simulink model "Simulation"  (R2025b)
settings: Solver=ode4  StartTime=0.0  StopTime=Tfin  FixedStep=Ts  RelTol=1e-3
undefined symbols (not defined in the file): period, radius, ReferenceTypeNumber, speed, Ts
settings Model: SimulationMode=accelerator  SILPILSystemUnderTest=refmodels  CodeVerificationMode=processor-in-the-loop (pil)  Creator=baldo  LastModifiedBy=robyd
settings OptimizationCC: DefaultParameterBehavior=Inlined  EnhancedBackFolding=on  PassReuseOutputArgsThreshold=0.0  OptimizeBlockOrder=speed  DifferentSizesBufferReuse=on  OptimizationCustomize=off
settings DebuggingCC: ParameterTunabilityLossMsg=error  UnconnectedInputMsg=warning  UnconnectedOutputMsg=warning  UnconnectedLineMsg=warning
settings ModelReferenceCC: EnableRefExpFcnMdlSchedulingChecks=on  PropagateVarSize=During execution
settings SFSimCC: MATLABDynamicMemAlloc=off
settings RTWCC: GPUComputeCapability=3.5  DLArmComputeVersion=19.05
settings CodeAppCC: ForceParamTrailComments=on  OperatorAnnotations=on

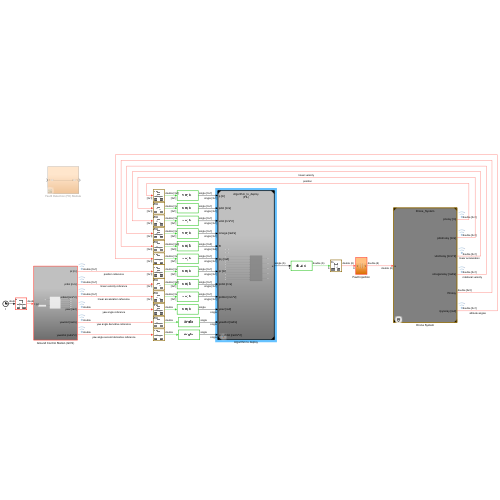
[thumbnail: Simulink's stored preview of the top-level diagram]
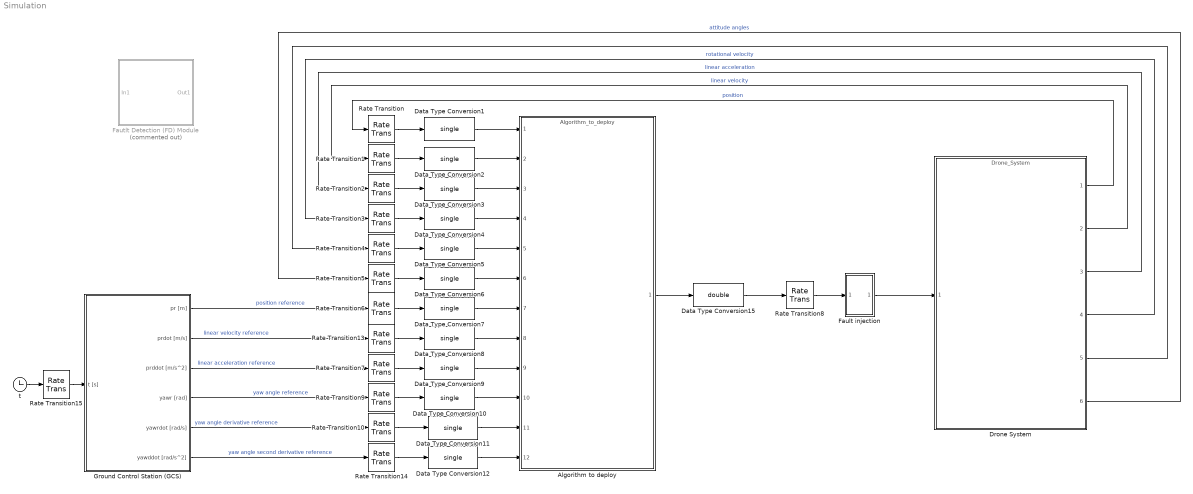
== system Simulation ==
  Algorithm to deploy : ModelReference  ModelNameDialog=Algorithm_to_deploy  SimulationMode=Processor-in-the-loop (PIL)  ModelReferenceVersion=9.14
  Data Type Conversion{1..12} (12 alike) : DataTypeConversion  OutDataTypeStr=single  SaturateOnIntegerOverflow=off  RndMeth=Floor
  Data Type Conversion15 : DataTypeConversion  OutDataTypeStr=double  SaturateOnIntegerOverflow=off  RndMeth=Floor
  Drone System : ModelReference  ModelNameDialog=Drone_System  ModelReferenceVersion=9.10  CopyOfModelProtected=on
  Fault injection : Subsystem
  Fautlt Detection (FD) Module : Subsystem  Commented=on
  Ground Control Station (GCS) : Subsystem
  Rate Transition{,1..7,9..10,13..14} (12 alike) : RateTransition  OutPortSampleTime=Ts_hw
  Rate Transition15 : RateTransition  OutPortSampleTime=Ts
  Rate Transition8 : RateTransition  OutPortSampleTime=Ts
  t : Clock
  wires:
  Algorithm to deploy/1 -> Data Type Conversion15/1
  Rate Transition/1 -> Data Type Conversion1/1
  Rate Transition1/1 -> Data Type Conversion2/1
  Rate Transition2/1 -> Data Type Conversion3/1
  Rate Transition3/1 -> Data Type Conversion4/1
  Rate Transition4/1 -> Data Type Conversion5/1
  Rate Transition5/1 -> Data Type Conversion6/1
  Rate Transition6/1 -> Data Type Conversion7/1
  Rate Transition13/1 -> Data Type Conversion8/1
  Rate Transition7/1 -> Data Type Conversion9/1
  Rate Transition9/1 -> Data Type Conversion10/1
  Rate Transition10/1 -> Data Type Conversion11/1
  Rate Transition14/1 -> Data Type Conversion12/1
  t/1 -> Rate Transition15/1
  Ground Control Station (GCS)/1(pr [m]) -> Rate Transition6/1  "position reference"
  Ground Control Station (GCS)/2(prdot [m/s]) -> Rate Transition13/1  "linear velocity reference"
  Ground Control Station (GCS)/3(prddot [m/s^2]) -> Rate Transition7/1  "linear acceleration reference"
  Ground Control Station (GCS)/4(yawr [rad]) -> Rate Transition9/1  "yaw angle reference"
  Ground Control Station (GCS)/5(yawrdot [rad/s]) -> Rate Transition10/1  "yaw angle derivative reference"
  Ground Control Station (GCS)/6(yawddot [rad/s^2]) -> Rate Transition14/1  "yaw angle second derivative reference"
  Data Type Conversion1/1 -> Algorithm to deploy/1
  Data Type Conversion2/1 -> Algorithm to deploy/2
  Data Type Conversion3/1 -> Algorithm to deploy/3
  Data Type Conversion4/1 -> Algorithm to deploy/4
  Data Type Conversion5/1 -> Algorithm to deploy/5
  Data Type Conversion6/1 -> Algorithm to deploy/6
  Data Type Conversion7/1 -> Algorithm to deploy/7
  Data Type Conversion8/1 -> Algorithm to deploy/8
  Data Type Conversion9/1 -> Algorithm to deploy/9
  Data Type Conversion10/1 -> Algorithm to deploy/10
  Data Type Conversion11/1 -> Algorithm to deploy/11
  Data Type Conversion12/1 -> Algorithm to deploy/12
  Data Type Conversion15/1 -> Rate Transition8/1
  Rate Transition15/1 -> Ground Control Station (GCS)/1(t [s])
  Drone System/1 -> Rate Transition/1  "position"
  Drone System/2 -> Rate Transition1/1  "linear velocity"
  Drone System/3 -> Rate Transition2/1  "linear acceleration"
  Drone System/4 -> Rate Transition3/1  "rotational velocity"
  Drone System/5 -> Rate Transition4/1
  Drone System/6 -> Rate Transition5/1  "attitude angles"
  Rate Transition8/1 -> Fault injection/1(In1)
  Fault injection/1(Out1) -> Drone System/1

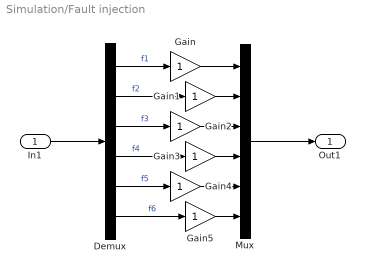
== system Simulation/Fault injection ==
  In1 : Inport
  Demux : Demux  Outputs=6
  Gain{,1..5} (6 alike) : Gain
  Mux : Mux  Inputs=6
  Out1 : Outport
  wires:
  Demux/2 -> Gain1/1  "f2"
  Demux/1 -> Gain/1  "f1"
  Demux/5 -> Gain4/1  "f5"
  Demux/3 -> Gain2/1  "f3"
  Gain5/1 -> Mux/6
  Gain2/1 -> Mux/3
  In1/1 -> Demux/1
  Mux/1 -> Out1/1
  Gain/1 -> Mux/1
  Demux/4 -> Gain3/1  "f4"
  Gain1/1 -> Mux/2
  Demux/6 -> Gain5/1  "f6"
  Gain4/1 -> Mux/5
  Gain3/1 -> Mux/4

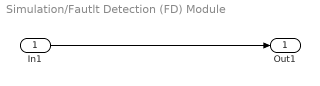
== system Simulation/Fautlt Detection (FD) Module ==
  In1 : Inport
  Out1 : Outport
  wires:
  In1/1 -> Out1/1

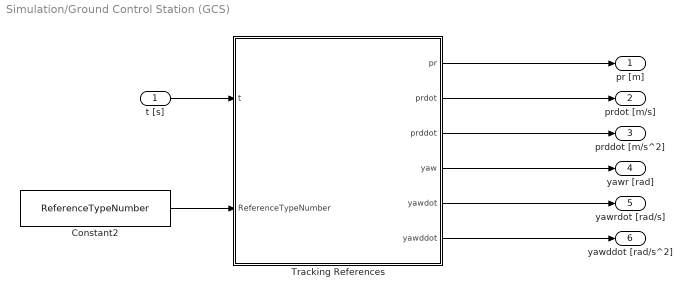
== system Simulation/Ground Control Station (GCS) ==
  t [s] : Inport
  Constant2 : Constant  Value=ReferenceTypeNumber  SampleTime=Ts
  Tracking References : MATLAB Function  TreatAsAtomicUnit=on
  pr [m] : Outport
  prdot [m/s] : Outport  Port=2
  prddot [m/s^2] : Outport  Port=3
  yawr [rad] : Outport  Port=4
  yawrdot [rad/s] : Outport  Port=5
  yawddot [rad/s^2] : Outport  Port=6
  wires:
  Tracking References/5(yawdot) -> yawrdot [rad/s]/1
  Tracking References/6(yawddot) -> yawddot [rad/s^2]/1
  Tracking References/3(prddot) -> prddot [m/s^2]/1
  Tracking References/2(prdot) -> prdot [m/s]/1
  Tracking References/4(yaw) -> yawr [rad]/1
  Tracking References/1(pr) -> pr [m]/1
  t [s]/1 -> Tracking References/1(t)
  Constant2/1 -> Tracking References/2(ReferenceTypeNumber)

== matlab function Simulation/Ground Control Station (GCS)/Tracking References ==
  data: t input; pr output; prdot output; prddot output; yaw output; speed parameter; period parameter; radius parameter; ReferenceTypeNumber input; yawdot output; yawddot output
function [pr,prdot,prddot,yaw,yawdot,yawddot] = RefGen(t, speed, period, radius, ReferenceTypeNumber)

% Extended references with derivatives
% prExtended = [pr prdot prddot] in R^{3x3}
% yawExtended = [yaw yawdot yawddot] in R^{1x3}

r = radius;
T = period;
v = speed;

if ReferenceTypeNumber == 0  % Origin

    prExtended = [NullWaveExtended(t); NullWaveExtended(t); NullWaveExtended(t)];
    yawExtended = NullWaveExtended(t);

elseif ReferenceTypeNumber == 1  % Constant speed in direction of xE

    prExtended = [speed*rampExtended(t); NullWaveExtended(t); NullWaveExtended(t)];
    yawExtended = NullWaveExtended(t);

elseif ReferenceTypeNumber == 2  % Constant speed in direction of yE

    prExtended = [NullWaveExtended(t); speed*rampExtended(t); NullWaveExtended(t)];
    yawExtended = NullWaveExtended(t);

elseif ReferenceTypeNumber == 3  % Constant speed in direction of -zE

    prExtended = [NullWaveExtended(t); NullWaveExtended(t); -speed*rampExtended(t)];
    yawExtended = NullWaveExtended(t);

elseif ReferenceTypeNumber == 4  % Ascending spiral
    
    pulsation = 2*pi/period;
    prExtended = [radius*CosineWaveExtended(t,pulsation)-radius*[1 0 0]; radius*SineWaveExtended(t,pulsation); -speed*rampExtended(t)];
    yawExtended = zeros(1,3);

    % omegayaw = 2*pi/5;
    % yawExtended = SineWaveExtended(t,omegayaw);

elseif ReferenceTypeNumber == 5  % Ascending 8-shape

    pulsation = 2*pi/period;
    prExtended = [radius*CosineWaveExtended(t,pulsation)-radius*[1 0 0]; 0.5*radius*SineWaveExtended(t,2*pulsation); -speed*rampExtended(t)];
    yawExtended = zeros(1,3);

elseif ReferenceTypeNumber == 6  % Square around e3

    prExtended = zeros(3,3);
    yawExtended = zeros(1,3);
    
    % L = 2*r;
    % t2 = mod(t,T);
    % pr = (4*L/T)*[ramp(t2)-ramp(t2-T/4)-ramp(t2-T/2)+ramp(t2-3*T/4); ramp(t2-T/4)-ramp(t2-T/2)-ramp(t2-3*T/4)+ramp(t2-T); -v*t];
    % psir = 0;
elseif ReferenceTypeNumber == 7

    prExtended = [SawtoothWaveExtended(t,20); NullWaveExtended(t); NullWaveExtended(t)];
    yawExtended = zeros(1,3);

elseif ReferenceTypeNumber == 8
    
    prExtended = [NullWaveExtended(t); NullWaveExtended(t); -SawtoothWave(t,20) 0 0];
    yawExtended = zeros(1,3);

elseif ReferenceTypeNumber == 9  % Descending spiral
    
    pulsation = 2*pi/period;
    prExtended = [radius*CosineWaveExtended(t,pulsation)-radius*[1 0 0]; 0.5*radius*SineWaveExtended(t,2*pulsation); (speed/2)*rampExtended(t)];
    yawExtended = zeros(1,3);

elseif ReferenceTypeNumber == 10  % Descending 8-shape

    pulsation = 2*pi/period;
    prExtended = [radius*CosineWaveExtended(t,pulsation)-radius*[1 0 0]; radius*SineWaveExtended(t,2*pulsation); (speed/2)*rampExtended(t)];
    yawExtended = zeros(1,3);

else
    error('ReferenceType non supported.')
    prExtended = zeros(3,3);
    yawExtended = zeros(1,3);
end

pr = prExtended(:,1);
prdot = prExtended(:,2);
prddot = prExtended(:,3);
yaw = yawExtended(1);
yawdot = yawExtended(2);
yawddot = yawExtended(3);

end
%%%%%%%%%%%%%%%%%%%%%%%%%%%%%%%%%%%
%         Basic signals           %
%%%%%%%%%%%%%%%%%%%%%%%%%%%%%%%%%%%
function u = NullWave(t)
    u = 0;
end
function u = step(t)
    if t >= 0
        u = 1;
    else
        u = 0;
    end
end
function u = ramp(t)
    u = t*step(t);
end
function u = SquareWave(t,T)
    t = mod(t,T);
    u = step(t)-step(t-T/2);
end
function u = SawtoothWave(t,T)
    t = mod(t,T);
    u = ramp(t)-2*ramp(t-T/2);
end
function u = SineWave(t,omega)
    u = sin(omega*t);
end
function u = CosineWave(t,omega)
    u = cos(omega*t);
end
%%%%%%%%%%%%%%%%%%%%%%%%%%%%%%%%%%%
%    Signals with derivatives     %
%%%%%%%%%%%%%%%%%%%%%%%%%%%%%%%%%%%
function uExtended = NullWaveExtended(t)
    uExtended = [0 0 0];
end
function uExtended = stepExtended(t)
    u = step(t);
    udot = 0;
    uddot = 0;
    uExtended = [u udot uddot];
end
function uExtended = rampExtended(t)
    u = ramp(t);
    udot = step(t);
    uddot = 0;
    uExtended = [u udot uddot];
end
function uExtended = SquareWaveExtended(t,T)
    t = mod(t,T);
    u = step(t)-step(t-T/2);
    udot = 0;
    uddot = 0;
    uExtended = [u udot uddot];
end
function uExtended = SawtoothWaveExtended(t,T)
    t = mod(t,T);
    u = ramp(t)-2*ramp(t-T/2);
    udot = step(t) - 2*step(t-T/2);
    uddot = 0;
    uExtended = [u udot uddot];
end
function uExtended = SineWaveExtended(t,omega)
    uExtended = [SineWave(t,omega) omega*CosineWave(t,omega) -(omega^2)*SineWave(t,omega)];
end
function uExtended = CosineWaveExtended(t,omega)
    uExtended = [CosineWave(t,omega) -omega*SineWave(t,omega) -(omega^2)*CosineWave(t,omega)];
end
